simulink model "battery_synthetic"  (R2017a)
settings: Solver=FixedStepAuto  StartTime=0.0  StopTime=36257  FixedStep=1  MaxStep=0.1  RelTol=1e-4  EnableMultiTasking=on
undefined symbols (not defined in the file or in its folder): Cadmium, Nickel
libraries: powerlib x3, electricdrivelib x1
Description:
  | Copyright 2008-2017 The MathWorks, Inc.
settings Model: Creator=MathWorks  LastModifiedBy=root
settings DataIOCC: LimitDataPoints=on  SaveFormat=Array  SignalLoggingSaveFormat=ModelDataLogs
settings OptimizationCC: ExpressionDepthLimit=2147483647  InitFltsAndDblsToZero=on  LifeSpan=inf
settings DebuggingCC: UnderspecifiedInitializationDetection=Classic  MergeDetectMultiDrivingBlocksExec=none  SignalResolutionControl=TryResolveAllWithWarning  SolverPrmCheckMsg=warning  FcnCallInpInsideContextMsg=warning  AllowSymbolicDim=off  StateNameClashWarn=warning  SFUnexpectedBacktrackingDiag=warning  SFNoUnconditionalDefaultTransitionDiag=warning  SFExecutionAtInitializationDiag=none
settings HardwareCC: ProdBitPerPointer=32  ProdBitPerSizeT=32  ProdBitPerPtrDiffT=32  ProdLargestAtomicFloat=None  ProdIntDivRoundTo=Undefined  ProdEndianess=Unspecified  ProdWordSize=32  ProdHWDeviceType=32-bit Generic
settings ModelReferenceCC: UpdateModelReferenceTargets=Force  PropagateSignalLabelsOutOfModel=off
settings GRTTargetCC: TargetLangStandard=C89/C90 (ANSI)  GeneratePreprocessorConditionals=Disable all  CombineOutputUpdateFcns=off  GRTInterface=on
settings ConfigComp: CovMetricSettings=dw  CovHtmlReporting=on  CovSaveCumulativeToWorkspaceVar=on  CovSaveSingleToWorkspaceVar=on  CovExternalEMLEnable=off

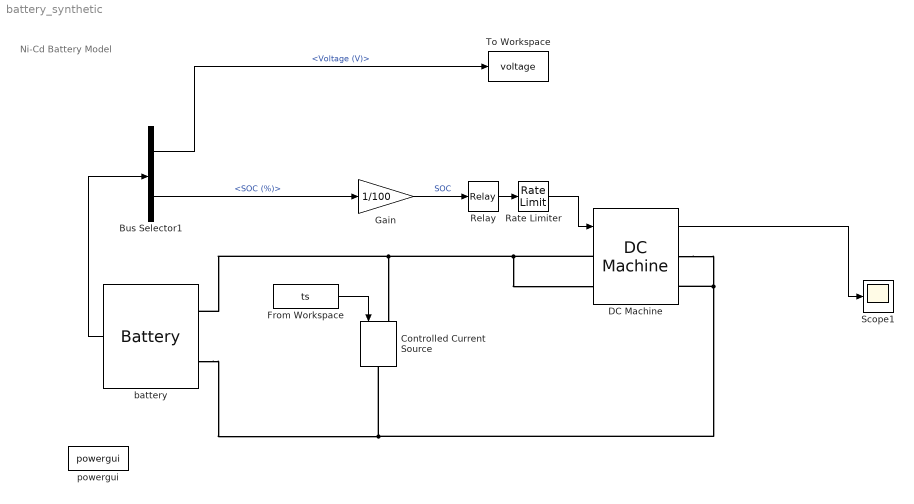
== system battery_synthetic ==
  note: Ni-Cd Battery Model
  Bus Selector1 : BusSelector  OutputSignals=Voltage (V),SOC (%)
  Controlled Current Source : powerlib/Electrical Sources/Controlled Current Source  Initialize=on  Source_Type=AC  Amplitude=0  Phase=0  Frequency=0  Measurements=None
  DC Machine : powerlib/Machines/DC Machine  PresetModel=No  MechanicalLoad=Torque TL  FieldType=Wound  ShowDetailedParameters=on  MeasurementBus=off  RLa=[0.4832 0.006763]  RLf=[84.91 13.39]  Laf=0.7096  MachineConstant=Torque constant (N.m/A)  Ke=1.8  Kt=1.8  J=0.2053  Bm=0.007032  Tf=0  w0=0  Ifinit=0  TsPowergui=0  TsBlock=-1
  From Workspace : FromWorkspace  VariableName=ts  SampleTime=0
  Gain : Gain  Gain=1/100
  Rate Limiter : RateLimiter  RisingSlewLimit=100  FallingSlewLimit=-100
  Relay : Relay  OnSwitchValue=0.8  OffSwitchValue=0.4  OnOutputValue=0  OffOutputValue=-200
  Scope1 : Scope
  To Workspace : ToWorkspace  VariableName=voltage  SaveFormat=Timeseries  SampleTime=-1
  battery : electricdrivelib/Extra Sources/Battery  BatType=Nickel-Cadmium  ShowTempParam=off  ThermalPreset=no  ShowAgeParam=on  NomV=27  NomQ=340  SOC=100  Batt_Tr=30  PresetModel=on  MaxQ=386.3636  MinV=20.25  FullV=30.8927  Dis_rate=68  R=0.00079412  Normal_OP=326.8636  expZone="[28.8106      95.0455]"  current=50  Units=Ampere-hour  Tci=20  NomT=25  T2=0  MaxQ2=2.208  FullV2=3.45  Normal_OP2=2.8  expZone2="[3.22        0.23]"  Rca=0.6  ti=1000  Dp=0  Neq0=0  Tsim=1e6  Ta1=25  Qeol=5.4*0.9  Reol=0.013333*1.2  Char_age=[2.3478, 3]  Dis_age=[2.3478, 10]  N1=1500  N2=10500  N3=1000  N4=1400  Ta2=45  N5=950
  powergui : powerlib/powergui  SimulationMode=Discrete  SampleTime=1  frequency=60  Iterations=50  frequencyindice=0  Pbase=100e6  ErrMax=1e-4  UnitsV=kV  UnitsW=MW  buscounter=0  FunctionMessages=off  echomessages=off  EnableUseOfTLC=off  CurrentSourceSwitches=off  DisableSnubberDevices=off  DisableRonSwitches=off  DisableVfSwitches=off  DisplayEquations=off  SolverType=Tustin/Backward Euler (TBE)  Interpol=off  ExternalGateDelay=off  methode=off  Ts=100  x0status=blocks  SPID=off  SwTol=0  HookPort=off  RestoreLinks=warning  ResistiveCurrentMeasurement=off  Frange=[0:2:500]  Ylog=off  Xlog=on  ShowGrid=off  save=off  variable=ZData  structure=0  ZoomFFT=on  StartTime=0.0  cycles=1  DisplayStyle=1  fundamental=60  FreqAxis=off  MaxFrequency=1000  frequencyindicesteady=1  RmsSteady=1  display=off
  wires:
  Relay/1 -> Rate Limiter/1
  Rate Limiter/1 -> DC Machine/1
  battery/1 -> Bus Selector1/1
  Bus Selector1/2 -> Gain/1  "<SOC (%)>"
  Gain/1 -> Relay/1  "SOC"
  From Workspace/1 -> Controlled Current Source/1
  Bus Selector1/1 -> To Workspace/1  "<Voltage (V)>"
  DC Machine/1 -> Scope1/1
  connections:
  battery/LConn2 -- DC Machine/RConn1 -- DC Machine/RConn2 -- Controlled Current Source/RConn1
  battery/LConn1 -- DC Machine/LConn1 -- DC Machine/LConn2 -- Controlled Current Source/LConn1
